simulink model "simulink_example"  (R2014b)
settings: Solver=FixedStepDiscrete  StartTime=0.0  StopTime=inf  FixedStep=1/100  RelTol=1e-3
libraries: simulink x1, PaPI x1
settings Model: Creator=sven  LastModifiedBy=sven
settings OptimizationCC: OptimizeModelRefInitCode=on  LifeSpan=Inf
settings DebuggingCC: UnderspecifiedInitializationDetection=Classic  MergeDetectMultiDrivingBlocksExec=none  InheritedTsInSrcMsg=none  StateNameClashWarn=warning
settings RTWCC: SystemTargetFile=ert_linux.tlc  MakeCommand="make_rtw OPTS=\"-DWITH_HW -std=gnu++11\""  TemplateMakefile=ert_linux.tmf  Description=Linux Embedded Coder  ProcessScript=ert_linux_make_rtw_hook  TargetLang=C++
settings CodeAppCC: IgnoreCustomStorageClasses=off
settings STFCustomTargetCC: ModelReferenceCompliant=off  CombineOutputUpdateFcns=on  ERTCustomFileBanners=on  SupportContinuousTime=off  SupportNonInlinedSFcns=off  MATLABClassNameForMDSCustomization=Simulink.SoftwareTarget.ERTCustomization  GRTInterface=off  SystemTargetFile=ert_linux.tlc
settings ERTTargetCC: ModelReferenceCompliant=off  ParMdlRefBuildCompliant=off  CompOptLevelCompliant=off  ConcurrentExecutionCompliant=off  ERTFirstTimeCompliant=off  ModelStepFunctionPrototypeControlCompliant=off  CPPClassGenCompliant=off  ExtMode=on  InlinedParameterPlacement=NonHierarchical  ERTCustomFileTemplate=ert_linux_file_process.tlc

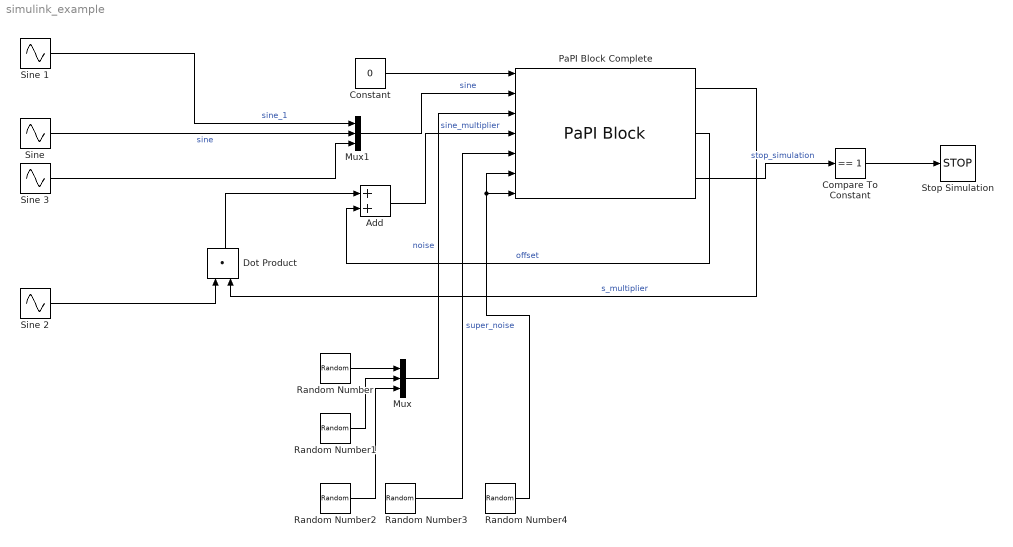
== system simulink_example ==
  Add : Sum
  Compare To Constant : simulink/Logic and Bit Operations/Compare To Constant  relop===  const=1  OutDataTypeStr=boolean
  Constant : Constant  Value=0  OutDataTypeStr=int32
  Dot Product : DotProduct  InputSameDT=on  OutDataTypeStr=Inherit: Inherit via internal rule
  Mux : Mux  Inputs=3
  Mux1 : Mux  Inputs=3
  PaPI Block Complete : PaPI/PaPI Block  amount_parameters=[1,1,1]  define_inputs=[3,3,1,300,2000,2000]  split_inputs=[1,1,1,0,0,0]  json_string='{}'  use_external_file=on  external_file='./simulink_example_config.json'  UDPLocalPort=20001  UDPRemotePort=20000  UDPRemoteIP='127.0.0.1'  UDPStart=on  sampleTime=-1
  Random Number : RandomNumber  Variance=2  SampleTime=0.1
  Random Number1 : RandomNumber  Variance=3  SampleTime=0.1
  Random Number2 : RandomNumber  Variance=4  SampleTime=0.1
  Random Number3 : RandomNumber  Mean=ones(1,300)  Variance=ones(1,300)*4  Seed=linspace(1,300,300)  SampleTime=0.1  VectorParams1D=off
  Random Number4 : RandomNumber  Mean=ones(1,2000)  Variance=ones(1,2000)*4  Seed=linspace(1,2000,2000)  SampleTime=0.1  VectorParams1D=off
  Sine : Sin  Amplitude=5
  Sine 1 : Sin  Amplitude=3
  Sine 2 : Sin  Amplitude=0.1  Frequency=2
  Sine 3 : Sin  Amplitude=3  Frequency=5
  Stop Simulation : Stop
  wires:
  PaPI Block Complete/1 -> Dot Product/2  "s_multiplier"
  Sine 2/1 -> Dot Product/1
  Random Number/1 -> Mux/1
  Random Number1/1 -> Mux/2
  Random Number2/1 -> Mux/3
  Sine 1/1 -> Mux1/1  "sine_1"
  Sine 3/1 -> Mux1/3
  Mux1/1 -> PaPI Block Complete/2  "sine"
  Mux/1 -> PaPI Block Complete/3  "noise"
  Sine/1 -> Mux1/2  "sine"
  Random Number3/1 -> PaPI Block Complete/5  "super_noise"
  Constant/1 -> PaPI Block Complete/1
  Add/1 -> PaPI Block Complete/4  "sine_multiplier"
  Dot Product/1 -> Add/1
  PaPI Block Complete/2 -> Add/2  "offset"
  PaPI Block Complete/3 -> Compare To Constant/1  "stop_simulation"
  Compare To Constant/1 -> Stop Simulation/1
  Random Number4/1 -> PaPI Block Complete/7, PaPI Block Complete/6
